simulink library "clc_closed_loop_controller_lib"  (R2016b)
settings: Solver=ode45  StartTime=0.0  StopTime=10.0  RelTol=1e-3  EnableMultiTasking=on
values from neighbouring files (symbols this model uses):
  ctl_ts = astrobee_fsw_step_size    [ctl_controller_init.m]
undefined symbols (not defined in the file or in its folder): DiscIntNeverNeededParam, tun_accel_gain, tun_alpha_gain, tun_ctl_att_sat_lower, tun_ctl_att_sat_upper, tun_ctl_linear_force_limit, tun_ctl_pos_sat_lower, tun_ctl_pos_sat_upper
libraries: simulink x6, math_utils x5, clc_closed_loop_controller_lib x1
settings Model: Creator=jfusco1  LastModifiedBy=jfusco1
settings DataIOCC: LimitDataPoints=on  SaveFormat=Array
settings OptimizationCC: LifeSpan=inf
settings DebuggingCC: AllowSymbolicDim=off  SFUnexpectedBacktrackingDiag=warning  SFNoUnconditionalDefaultTransitionDiag=warning  SFExecutionAtInitializationDiag=none
settings HardwareCC: ProdBitPerPointer=32  ProdBitPerSizeT=32  ProdBitPerPtrDiffT=32  ProdLargestAtomicFloat=None  ProdIntDivRoundTo=Undefined  ProdEndianess=Unspecified  ProdWordSize=32  ProdHWDeviceType=32-bit Generic
settings ModelReferenceCC: PropagateSignalLabelsOutOfModel=off
settings GRTTargetCC: TargetLangStandard=C89/C90 (ANSI)  GeneratePreprocessorConditionals=Disable all
settings ConfigComp: CovMetricSettings=dw  CovHtmlReporting=on  CovSaveCumulativeToWorkspaceVar=on  CovSaveSingleToWorkspaceVar=on  CovExternalEMLEnable=off

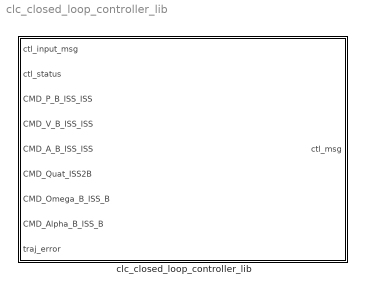
== system clc_closed_loop_controller_lib ==
  clc_closed_loop_controller_lib : Subsystem

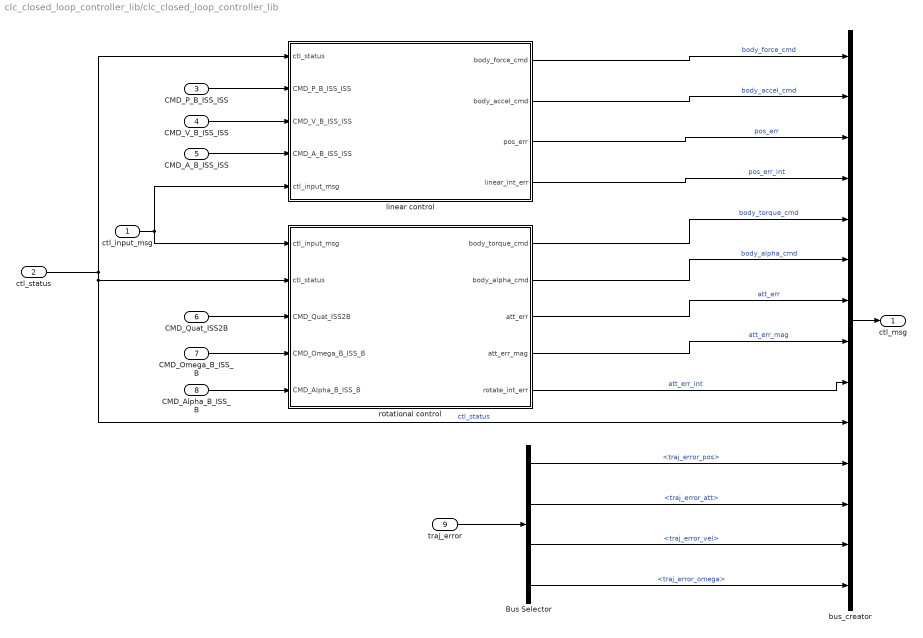
== system clc_closed_loop_controller_lib/clc_closed_loop_controller_lib ==
  ctl_input_msg : Inport  OutDataTypeStr=Bus: ctl_input_msg
  ctl_status : Inport  Port=2
  CMD_P_B_ISS_ISS : Inport  Port=3
  CMD_V_B_ISS_ISS : Inport  Port=4
  CMD_A_B_ISS_ISS : Inport  Port=5
  CMD_Quat_ISS2B : Inport  Port=6
  CMD_Omega_B_ISS_B : Inport  Port=7
  CMD_Alpha_B_ISS_B : Inport  Port=8
  traj_error : Inport  Port=9
  Bus Selector : BusSelector  OutputSignals=traj_error_pos,traj_error_att,traj_error_vel,traj_error_omega
  bus_creator : BusCreator  Inputs=14  OutDataTypeStr=Bus: ctl_msg  NonVirtualBus=on
  linear control : Subsystem
  rotational control : Subsystem
  ctl_msg : Outport
  wires:
  Bus Selector/4 -> bus_creator/14  "<traj_error_omega>"
  Bus Selector/1 -> bus_creator/11  "<traj_error_pos>"
  Bus Selector/3 -> bus_creator/13  "<traj_error_vel>"
  Bus Selector/2 -> bus_creator/12  "<traj_error_att>"
  traj_error/1 -> Bus Selector/1
  CMD_P_B_ISS_ISS/1 -> linear control/2(CMD_P_B_ISS_ISS)
  CMD_V_B_ISS_ISS/1 -> linear control/3(CMD_V_B_ISS_ISS)
  ctl_input_msg/1 -> rotational control/1(ctl_input_msg), linear control/5(ctl_input_msg)
  CMD_Quat_ISS2B/1 -> rotational control/3(CMD_Quat_ISS2B)
  CMD_Omega_B_ISS_B/1 -> rotational control/4(CMD_Omega_B_ISS_B)
  linear control/1(body_force_cmd) -> bus_creator/1  "body_force_cmd"
  linear control/3(pos_err) -> bus_creator/3  "pos_err"
  linear control/4(linear_int_err) -> bus_creator/4  "pos_err_int"
  rotational control/1(body_torque_cmd) -> bus_creator/5  "body_torque_cmd"
  rotational control/3(att_err) -> bus_creator/7  "att_err"
  rotational control/4(att_err_mag) -> bus_creator/8  "att_err_mag"
  rotational control/5(rotate_int_err) -> bus_creator/9  "att_err_int"
  ctl_status/1 -> bus_creator/10, rotational control/2(ctl_status), linear control/1(ctl_status)  "ctl_status"
  bus_creator/1 -> ctl_msg/1
  linear control/2(body_accel_cmd) -> bus_creator/2  "body_accel_cmd"
  rotational control/2(body_alpha_cmd) -> bus_creator/6  "body_alpha_cmd"
  CMD_A_B_ISS_ISS/1 -> linear control/4(CMD_A_B_ISS_ISS)
  CMD_Alpha_B_ISS_B/1 -> rotational control/5(CMD_Alpha_B_ISS_B)

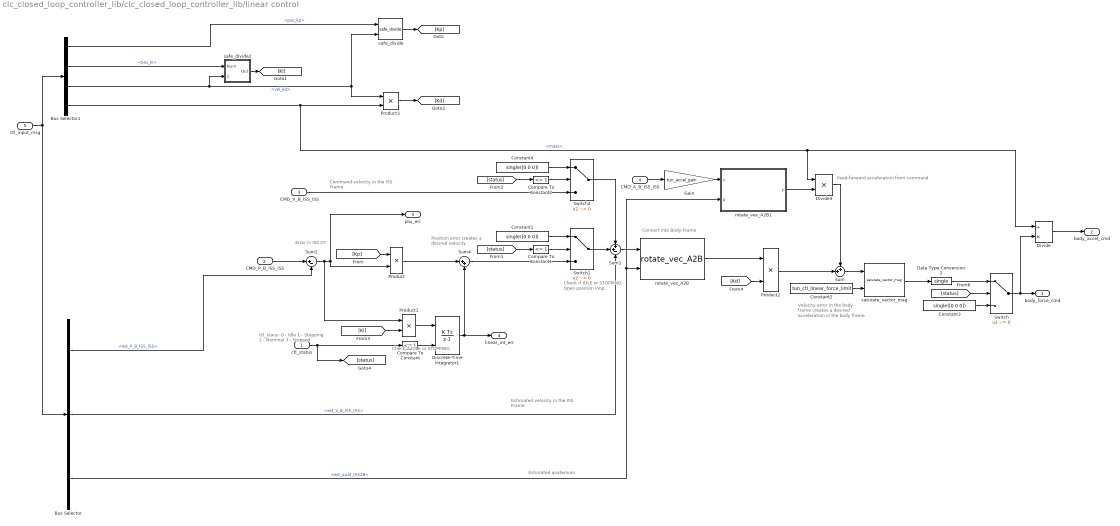
== system clc_closed_loop_controller_lib/clc_closed_loop_controller_lib/linear control ==
  note: Velocity error in the
      | body frame creates a
      | desired acceleration in
      | the body frame
  note: Position error
      | creates a desired
      | velocity
  note: Error in ISS CF
  note: Convert into Body Frame
  note: Command velocity in
      | the ISS Frame
  note: Estimated velocity in
      | the ISS Frame
  note: ctl_staus:
      | 0 - Idle
      | 1 - Stopping
      | 2 - Nominal
      | 3 - Stopped
  note: Check if IDLE or
      | STOPPING
  note: Check if IDLE or
      | STOPPING.
      | Open position
      | loop.
  note: Estimated quaternion
  note: Feed-forward acceleration from command
  ctl_status : Inport
  CMD_P_B_ISS_ISS : Inport  Port=2
  CMD_V_B_ISS_ISS : Inport  Port=3
  CMD_A_B_ISS_ISS : Inport  Port=4
  ctl_input_msg : Inport  Port=5  OutDataTypeStr=Bus: ctl_input_msg
  Bus Selector : BusSelector  OutputSignals=est_P_B_ISS_ISS,est_V_B_ISS_ISS,est_quat_ISS2B
  Bus Selector1 : BusSelector  OutputSignals=pos_kp,pos_ki,vel_kd,mass
  Compare To Constant : simulink/Logic and Bit Operations/Compare To Constant  relop=<=  const=1  OutDataTypeStr=boolean
  Compare To Constant1 : simulink/Logic and Bit Operations/Compare To Constant  relop=<=  const=1  OutDataTypeStr=boolean
  Compare To Constant2 : simulink/Logic and Bit Operations/Compare To Constant  relop=<=  const=1  OutDataTypeStr=boolean
  Constant1 : Constant  Value=single([0 0 0])
  Constant2 : Constant  Value=tun_ctl_linear_force_limit
  Constant3 : Constant  Value=single([0 0 0])
  Constant4 : Constant  Value=single([0 0 0])
  Data Type Conversion2 : DataTypeConversion  OutDataTypeStr=single
  Discrete-Time Integrator1 : DiscreteIntegrator  gainval=1  ExternalReset=level  InitialCondition=single([0 0 0])  InitialConditionSetting=State (most efficient)  SampleTime=ctl_ts  LimitOutput=on  UpperSaturationLimit=tun_ctl_pos_sat_upper  LowerSaturationLimit=tun_ctl_pos_sat_lower  ICPrevOutput=DiscIntNeverNeededParam  ICPrevScaledInput=DiscIntNeverNeededParam
      settings: AttributesFormatString=|
      | Gain: %<gainval>
      | Ts: %<SampleTime>
      | Upper Sat: %<UpperSaturationLimit>
      | Lower Sat: %<LowerSaturationLimit>
  Divide : Product  Inputs=/*
  Divide3 : Product  Inputs=**
  Gain : Gain  Gain=tun_accel_gain
  Product{,1..3} (4 alike) : Product
  Sum : Sum  Inputs=++|
  Sum1 : Sum  Inputs=++-
  Sum2 : Sum  Inputs=|+-
  Sum4 : Sum  Inputs=|++
  Switch : Switch  Criteria=u2 ~= 0
  Switch1 : Switch  Criteria=u2 ~= 0
  Switch2 : Switch  Criteria=u2 ~= 0
  rotate_vec_A2B : math_utils/rotate_vec_A2B  SystemSampleTime=-1
  rotate_vec_A2B1 : Subsystem
      mask Display:
      | disp('Rotate Vector\n\n')
      | disp('A to B');
  safe_divide : clc_closed_loop_controller_lib/clc_closed_loop_controller_lib/rotational control/safe_divide
  safe_divide2 : Subsystem
  saturate_vector_mag : math_utils/saturate_vector_mag  SystemSampleTime=-1
  body_force_cmd : Outport
  body_accel_cmd : Outport  Port=2
  pos_err : Outport  Port=3
  linear_int_err : Outport  Port=4
  wires:
  Switch/1 -> Divide/2, body_force_cmd/1
  Bus Selector/3 -> rotate_vec_A2B1/2(q), rotate_vec_A2B/2  "<est_quat_ISS2B>"
  [status] -> Switch/2
  saturate_vector_mag/1 -> Data Type Conversion2/1
  Constant2/1 -> saturate_vector_mag/2
  Product1/1 -> Discrete-Time Integrator1/1
  Discrete-Time Integrator1/1 -> linear_int_err/1, Sum4/2
  Product/1 -> Sum4/1
  Bus Selector/1 -> Sum2/2  "<est_P_B_ISS_ISS>"
  Sum2/1 -> Product/2, pos_err/1, Product1/1
  CMD_P_B_ISS_ISS/1 -> Sum2/1
  CMD_V_B_ISS_ISS/1 -> Switch2/3
  Bus Selector/2 -> Sum1/3  "<est_V_B_ISS_ISS>"
  rotate_vec_A2B/1 -> Product2/1
  Sum1/1 -> rotate_vec_A2B/1
  Constant3/1 -> Switch/3
  Data Type Conversion2/1 -> Switch/1
  ctl_status/1 -> Compare To Constant/1, [status]
  Compare To Constant/1 -> Discrete-Time Integrator1/2
  Switch1/1 -> Sum1/2
  Compare To Constant1/1 -> Switch1/2
  [status] -> Compare To Constant1/1
  Constant1/1 -> Switch1/1
  Sum4/1 -> Switch1/3
  Compare To Constant2/1 -> Switch2/2
  [status] -> Compare To Constant2/1
  Constant4/1 -> Switch2/1
  Switch2/1 -> Sum1/1
  Divide/1 -> body_accel_cmd/1
  [Kp] -> Product/1
  [Ki] -> Product1/2
  [Kd] -> Product2/2
  CMD_A_B_ISS_ISS/1 -> Gain/1
  Gain/1 -> rotate_vec_A2B1/1(v)
  rotate_vec_A2B1/1(y) -> Divide3/2
  Sum/1 -> saturate_vector_mag/1
  Product2/1 -> Sum/2
  Divide3/1 -> Sum/1
  safe_divide/1 -> [Kp]
  safe_divide2/1(Out) -> [Ki]
  Product3/1 -> [Kd]
  ctl_input_msg/1 -> Bus Selector1/1, Bus Selector/1
  Bus Selector1/4 -> Product3/2, Divide/1, Divide3/1  "<mass>"
  Bus Selector1/2 -> safe_divide2/1(Num)  "<pos_ki>"
  Bus Selector1/3 -> safe_divide2/2(Denom), Product3/1, safe_divide/2  "<vel_kd>"
  Bus Selector1/1 -> safe_divide/1  "<pos_kp>"

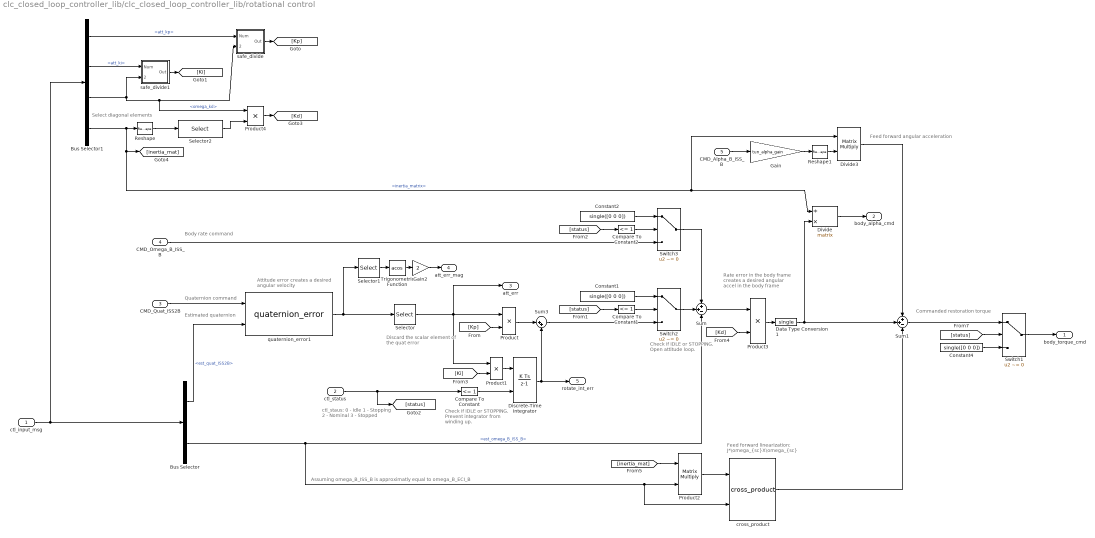
== system clc_closed_loop_controller_lib/clc_closed_loop_controller_lib/rotational control ==
  note: Rate error in the
      | body frame creates a
      | desired angular accel in
      | the body frame
  note: Attitude error creates a desired
      | angular velocity
  note: Discard the scalar
      | element of the quat error
  note: Body rate command
  note: Quaternion command
  note: Check if IDLE or
      | STOPPING.
      | Prevent
      | integrator from
      | winding up.
  note: ctl_staus:
      | 0 - Idle
      | 1 - Stopping
      | 2 - Nominal
      | 3 - Stopped
  note: Check if IDLE or
      | STOPPING.
      | Open attitude
      | loop.
  note: Estimated quaternion
  note: Feed forward linearization:
      | J*\omega_{sc}X\omega_{sc}
  note: Assuming omega_B_ISS_B is approximatly equal to omega_B_ECI_B
  note: Commanded restoration torque
  note: Select diagonal elements
  note: Feed forward angular acceleration
  ctl_input_msg : Inport  OutDataTypeStr=Bus: ctl_input_msg
  ctl_status : Inport  Port=2
  CMD_Quat_ISS2B : Inport  Port=3
  CMD_Omega_B_ISS_B : Inport  Port=4
  CMD_Alpha_B_ISS_B : Inport  Port=5
  Bus Selector : BusSelector  OutputSignals=est_quat_ISS2B,est_omega_B_ISS_B
  Bus Selector1 : BusSelector  OutputSignals=att_kp,att_ki,omega_kd,inertia_matrix
  Compare To Constant : simulink/Logic and Bit Operations/Compare To Constant  relop=<=  const=1  OutDataTypeStr=boolean
  Compare To Constant1 : simulink/Logic and Bit Operations/Compare To Constant  relop=<=  const=1  OutDataTypeStr=boolean
  Compare To Constant2 : simulink/Logic and Bit Operations/Compare To Constant  relop=<=  const=1  OutDataTypeStr=boolean
  Constant1 : Constant  Value=single([0 0 0])
  Constant2 : Constant  Value=single([0 0 0])
  Constant4 : Constant  Value=single([0 0 0])
  Data Type Conversion1 : DataTypeConversion  OutDataTypeStr=single
  Discrete-Time Integrator : DiscreteIntegrator  gainval=1  ExternalReset=level  InitialCondition=single([0 0 0])  InitialConditionSetting=State (most efficient)  SampleTime=ctl_ts  LimitOutput=on  UpperSaturationLimit=tun_ctl_att_sat_upper  LowerSaturationLimit=tun_ctl_att_sat_lower  ICPrevOutput=DiscIntNeverNeededParam  ICPrevScaledInput=DiscIntNeverNeededParam
      settings: AttributesFormatString=|
      | Gain: %<gainval>
      | Ts: %<SampleTime>
      | Upper Sat: %<UpperSaturationLimit>
      | Lower Sat: %<LowerSaturationLimit>
  Divide : Product  Inputs=/*  Multiplication=Matrix(*)
  Divide3 : Product  Inputs=**  Multiplication=Matrix(*)
  Gain : Gain  Gain=tun_alpha_gain
  Gain2 : Gain  Gain=2
  Product{,1,3..4} (4 alike) : Product
  Product2 : Product  Multiplication=Matrix(*)
  Reshape : Reshape  OutputDimensions=[21*21]
  Reshape1 : Reshape  OutputDimensionality=Column vector (2-D)
  Selector : Selector  InputPortWidth=4  IndexOptions=Index vector (dialog)  Indices=[1 2 3]  OutputSizes=1
  Selector1 : Selector  InputPortWidth=4  IndexOptions=Index vector (dialog)  Indices=[4]  OutputSizes=1
  Selector2 : Selector  InputPortWidth=9  IndexOptions=Index vector (dialog)  Indices=[1 5 9]  OutputSizes=1
  Sum : Sum  Inputs=++-
  Sum1 : Sum  Inputs=++-
  Sum3 : Sum  Inputs=|++
  Switch1 : Switch  Criteria=u2 ~= 0
  Switch2 : Switch  Criteria=u2 ~= 0
  Switch3 : Switch  Criteria=u2 ~= 0
  Trigonometric Function : Trigonometry  Operator=acos
  cross_product : math_utils/cross_product  SystemSampleTime=-1
  quaternion_error1 : math_utils/quaternion_error  SystemSampleTime=-1
  safe_divide : Subsystem
  safe_divide1 : Subsystem
  body_torque_cmd : Outport
  body_alpha_cmd : Outport  Port=2
  att_err : Outport  Port=3
  att_err_mag : Outport  Port=4
  rotate_int_err : Outport  Port=5
  wires:
  [status] -> Switch1/2
  ctl_status/1 -> Compare To Constant/1, [status]
  Product1/1 -> Discrete-Time Integrator/1
  Discrete-Time Integrator/1 -> rotate_int_err/1, Sum3/2
  Product/1 -> Sum3/1
  CMD_Omega_B_ISS_B/1 -> Switch3/3
  Bus Selector/2 -> Sum/3, cross_product/2, Product2/2  "<est_omega_B_ISS_B>"
  Bus Selector/1 -> quaternion_error1/2  "<est_quat_ISS2B>"
  Selector/1 -> Product/1, Product1/1, att_err/1
  CMD_Quat_ISS2B/1 -> quaternion_error1/1
  quaternion_error1/1 -> Selector1/1, Selector/1
  Product3/1 -> Data Type Conversion1/1
  Sum/1 -> Product3/1
  Compare To Constant/1 -> Discrete-Time Integrator/2
  Constant4/1 -> Switch1/3
  Compare To Constant1/1 -> Switch2/2
  [status] -> Compare To Constant1/1
  Constant1/1 -> Switch2/1
  Switch2/1 -> Sum/2
  Sum3/1 -> Switch2/3
  Trigonometric Function/1 -> Gain2/1
  Selector1/1 -> Trigonometric Function/1
  Gain2/1 -> att_err_mag/1
  Compare To Constant2/1 -> Switch3/2
  [status] -> Compare To Constant2/1
  Constant2/1 -> Switch3/1
  Switch3/1 -> Sum/1
  Product2/1 -> cross_product/1
  [inertia_mat] -> Product2/1
  Data Type Conversion1/1 -> Divide/2, Sum1/2
  Sum1/1 -> Switch1/1
  cross_product/1 -> Sum1/3
  Switch1/1 -> body_torque_cmd/1
  Divide/1 -> body_alpha_cmd/1
  safe_divide/1(Out) -> [Kp]
  Product4/1 -> [Kd]
  [Ki] -> Product1/2
  [Kd] -> Product3/2
  [Kp] -> Product/2
  ctl_input_msg/1 -> Bus Selector1/1, Bus Selector/1
  Bus Selector1/1 -> safe_divide/1(Num)  "<att_kp>"
  Bus Selector1/3 -> safe_divide1/2(Denom), Product4/1, safe_divide/2(Denom)  "<omega_kd>"
  Bus Selector1/2 -> safe_divide1/1(Num)  "<att_ki>"
  Bus Selector1/4 -> Reshape/1, [inertia_mat], Divide/1, Divide3/1  "<inertia_matrix>"
  Reshape/1 -> Selector2/1
  Selector2/1 -> Product4/2
  CMD_Alpha_B_ISS_B/1 -> Gain/1
  Gain/1 -> Reshape1/1
  Divide3/1 -> Sum1/1
  Reshape1/1 -> Divide3/2
  safe_divide1/1(Out) -> [Ki]

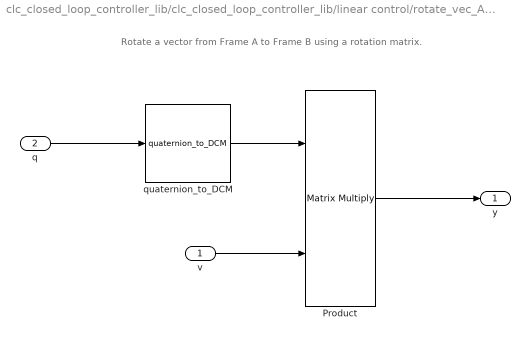
== system clc_closed_loop_controller_lib/clc_closed_loop_controller_lib/linear control/rotate_vec_A2B1 ==
  note: Rotate a vector from Frame A to Frame B using a rotation matrix.
  v : Inport
  q : Inport  Port=2  PortDimensions=4
  Product : Product  Multiplication=Matrix(*)
  quaternion_to_DCM : math_utils/quaternion_to_DCM  SystemSampleTime=-1
  y : Outport
  wires:
  q/1 -> quaternion_to_DCM/1
  quaternion_to_DCM/1 -> Product/1
  v/1 -> Product/2
  Product/1 -> y/1

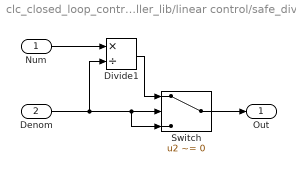
== system clc_closed_loop_controller_lib/clc_closed_loop_controller_lib/linear control/safe_divide2 ==
  Num : Inport
  Denom : Inport  Port=2
  Divide1 : Product  Inputs=*/
  Switch : Switch  Criteria=u2 ~= 0
  Out : Outport
  wires:
  Denom/1 -> Divide1/2, Switch/3, Switch/2
  Num/1 -> Divide1/1
  Divide1/1 -> Switch/1
  Switch/1 -> Out/1

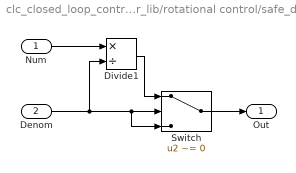
== system clc_closed_loop_controller_lib/clc_closed_loop_controller_lib/rotational control/safe_divide ==
  Num : Inport
  Denom : Inport  Port=2
  Divide1 : Product  Inputs=*/
  Switch : Switch  Criteria=u2 ~= 0
  Out : Outport
  wires:
  Denom/1 -> Divide1/2, Switch/3, Switch/2
  Num/1 -> Divide1/1
  Divide1/1 -> Switch/1
  Switch/1 -> Out/1

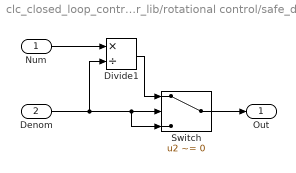
== system clc_closed_loop_controller_lib/clc_closed_loop_controller_lib/rotational control/safe_divide1 ==
  Num : Inport
  Denom : Inport  Port=2
  Divide1 : Product  Inputs=*/
  Switch : Switch  Criteria=u2 ~= 0
  Out : Outport
  wires:
  Switch/1 -> Out/1
  Divide1/1 -> Switch/1
  Num/1 -> Divide1/1
  Denom/1 -> Switch/2, Switch/3, Divide1/2
